simulink model "server"  (R2022b)
settings: Solver=FixedStepAuto  StartTime=0.0  StopTime=111111  FixedStep=0.1  RelTol=1e-3
settings Model: Creator=ROG  LastModifiedBy=ROG

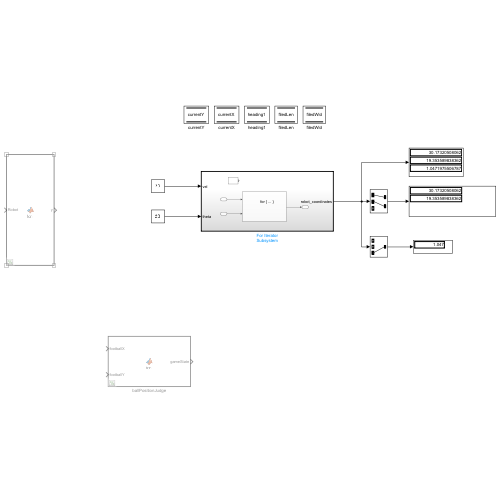
[thumbnail: Simulink's stored preview of the top-level diagram]
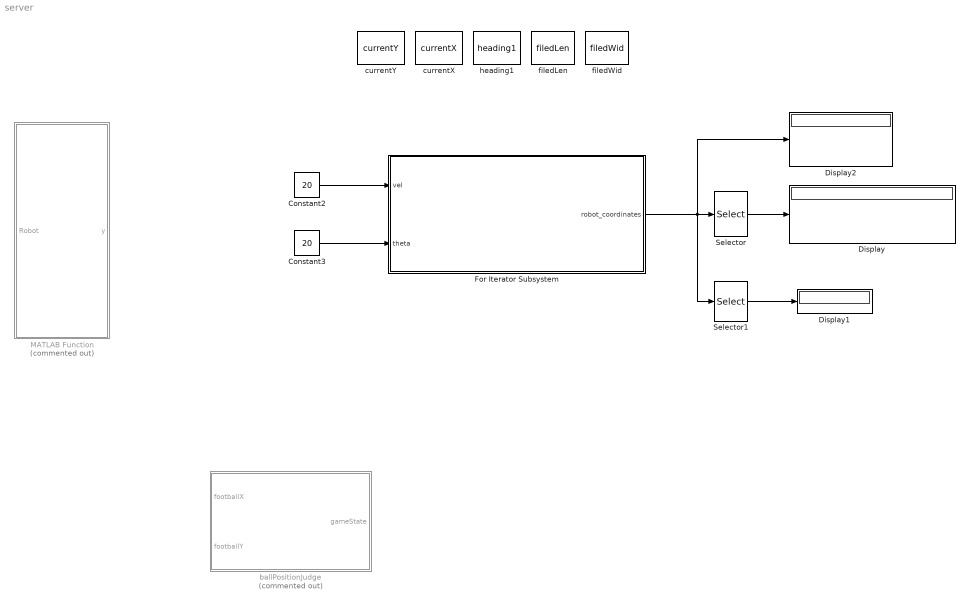
== system server ==
  Constant2 : Constant  Value=20
  Constant3 : Constant  Value=20
  Display : Display
  Display1 : Display
  Display2 : Display
  For Iterator Subsystem : Subsystem  TreatAsAtomicUnit=on
  MATLAB Function : MATLAB Function  Commented=on  TreatAsAtomicUnit=on
  Selector : Selector  InputPortWidth=3  IndexOptions=Index vector (dialog)  Indices=[1 2]  OutputSizes=1
  Selector1 : Selector  InputPortWidth=3  IndexOptions=Index vector (dialog)  Indices=[3]  OutputSizes=1
  ballPositionJudge : MATLAB Function  Commented=on  TreatAsAtomicUnit=on
  currentX : DataStoreMemory  DataStoreName=currentX  WriteAfterWriteMsg=warning  InitialValue=30  ShowAdditionalParam=off  OutMin=0  OutMax=60  OutDataTypeStr=double
  currentY : DataStoreMemory  DataStoreName=currentY  WriteAfterWriteMsg=warning  InitialValue=20  ShowAdditionalParam=off  OutMin=0  OutMax=90  OutDataTypeStr=double
  filedLen : DataStoreMemory  DataStoreName=filedLen  WriteAfterWriteMsg=warning  InitialValue=105  ShowAdditionalParam=off
  filedWid : DataStoreMemory  DataStoreName=filedWid  WriteAfterWriteMsg=warning  InitialValue=68  ShowAdditionalParam=off
  heading1 : DataStoreMemory  DataStoreName=heading1  WriteAfterWriteMsg=warning  InitialValue=pi  ShowAdditionalParam=off  OutDataTypeStr=double
  wires:
  Constant3/1 -> For Iterator Subsystem/2(theta)
  Constant2/1 -> For Iterator Subsystem/1(vel)
  For Iterator Subsystem/1(robot_coordinates) -> Selector1/1, Selector/1, Display2/1
  Selector/1 -> Display/1
  Selector1/1 -> Display1/1

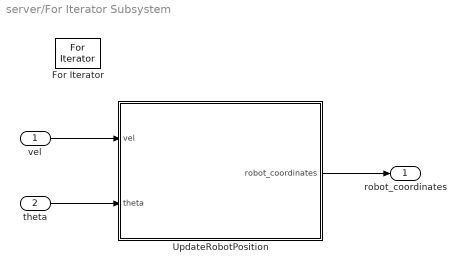
== system server/For Iterator Subsystem ==
  vel : Inport
  theta : Inport  Port=2
  For Iterator : ForIterator  IterationLimit=10  IterationVariableDataType=double
  UpdateRobotPosition : MATLAB Function  TreatAsAtomicUnit=on
  robot_coordinates : Outport
  wires:
  UpdateRobotPosition/1(robot_coordinates) -> robot_coordinates/1
  vel/1 -> UpdateRobotPosition/1(vel)
  theta/1 -> UpdateRobotPosition/2(theta)

== matlab function server/MATLAB Function ==
  data: Robot input; y output
function y = fcn(Robot)
    % properties
    currentX = Robot.currentPos(1);
    currentY = Robot.currentPos(2);
    currentHeading = Robot.currentPos(3);
    
y = Robot;

== matlab function server/ballPositionJudge ==
  data: footballX input; gameState output; footballY input
function gameState = fcn(footballX,footballY)
    global footballX;
    global footballY;
    global fieldLen;
    global fieldWid;
    % gameState : 1->normal, 0->out of boundary, 2->scored
%     global gameState;
    gameState = 1;
    
    if (footballX <= 0 && footballY > 30.34 && footballY < 37.66)
        % Away Team scored
        % Away Team socre + 1
        gameState = 2;
        
    elseif (footballX >= fieldLen && footballY > 30.34 && footballY < 37.66)
        % Our Team scored
        % Our Team socre + 1
        gameState = 2;

    elseif footballX < 0 || footballX > fieldLen || footballY < 0 || footballY > fieldWid
        % out of boundary
        gameState = 0;
    end
    
    if gameState == 1
        % normal play
    end    
end

== matlab function server/For Iterator Subsystem/UpdateRobotPosition ==
  data: vel input; robot_coordinates output; theta input; currentY data_store_memory; currentX data_store_memory; heading1 data_store_memory
function robot_coordinates  = UpdateRobotPosition(vel, theta)
    global currentX  currentY;  
    global heading1;
    % define sample time
    sampleTime = 0.01;

    % calculate the velocity vector of x, y
    velX = vel * cos(heading1);
    velY = vel * sin(heading1);

    % let heading in arrange [-pi, pi]
    
    % processing heading
    theta = theta / 2*pi;  % degree converted to pi
    if abs(theta) > pi/6
        heading1 = heading1 + pi/6;
    else
        heading1 = heading1 + theta;
    end

    if heading1 > pi
        heading1 = heading1 - 2 * pi;
    elseif heading1 < -pi
        heading1 = heading1 + 2 * pi;
    end

    % new position
    currentX = currentX + velX * sampleTime;
    currentY = currentY + velY * sampleTime;
    
    % put heading in vector
    currentPosition = [currentX, currentY, heading1];
    
   
    % output the vector
    robot_coordinates = currentPosition;
end
